simulink model "VendingMachine"  (R2020a)
settings: Solver=VariableStepAuto  StartTime=0.0  StopTime=100  RelTol=1e-3
libraries: simulink x1
settings Model: Creator=Hp  LastModifiedBy=Hp

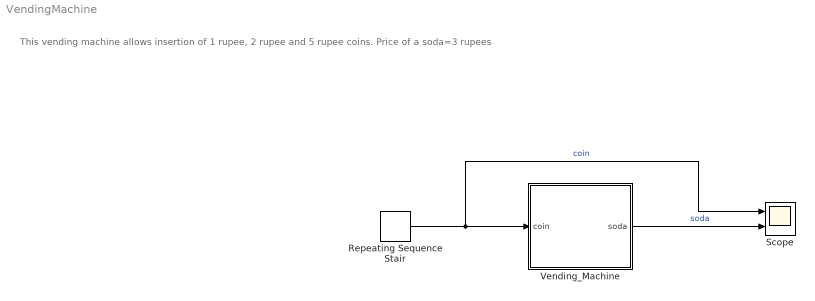
== system VendingMachine ==
  note: This vending machine allows insertion of 1 rupee, 2 rupee and 5 rupee coins.
      |
      | Price of a soda=3 rupees
  Repeating Sequence Stair : simulink/Sources/Repeating Sequence Stair  OutValues="[0 5 1 2 5 2 2 2 1 1  ].'"  tsamp=10  OutMin=[]  OutMax=[]  OutDataTypeStr=double  OutputDataTypeScalingMode=double  OutDataType=fixdt(0,8)  ConRadixGroup=Best Precision: Vector-wise  OutScaling=2^-12
  Scope : Scope  NumInputPorts=2
  Vending_Machine : Stateflow chart  TreatAsAtomicUnit=on
  wires:
  Repeating Sequence Stair/1 -> Scope/1, Vending_Machine/1(coin)  "coin"
  Vending_Machine/1(soda) -> Scope/2  "soda"

== stateflow chart VendingMachine/Vending_Machine ==
  state NoCoins
  state Got_1rupee
  state Got_2rupee
  (default) -> NoCoins
  NoCoins -> Got_1rupee [order 1] : [coin==1]{soda=0;}
  Got_1rupee -> NoCoins [order 2] : [coin==2]{soda=1;}
  Got_1rupee -> NoCoins [order 3] : [coin==5]{soda=2;}
  Got_1rupee -> Got_2rupee [order 1] : [coin==1]{soda=0;}
  Got_2rupee -> Got_1rupee [order 1] : [coin==2]{soda=1;}
  Got_2rupee -> Got_1rupee [order 3] : [coin==5]{soda=2;}
  Got_2rupee -> NoCoins [order 2] : [coin==1]{soda=1;}
  NoCoins -> Got_2rupee [order 3] : [coin==5]{soda=1;}
  NoCoins -> Got_2rupee [order 2] : [coin==2]{soda=0;}
  data: coin input; soda output
